simulink model "chap6_6sim"  (Simulink 7.7)
settings: Solver=ode45  StartTime=0.0  StopTime=10.0  RelTol=1e-3
settings Model: Creator=Administrator  LastModifiedBy=ljk
settings DataIOCC: SignalLoggingName=sigsOut
settings OptimizationCC: InitFltsAndDblsToZero=on
settings DebuggingCC: SaveWithParameterizedLinksMsg=none  SignalResolutionControl=TryResolveAllWithWarning  SolverPrmCheckMsg=none  MultiTaskDSMMsg=warning  MultiTaskCondExecSysMsg=none  StrictBusMsg=Warning
settings HardwareCC: TargetUnknown=on
settings RTWCC: IncludeERTFirstTime=on
settings GRTTargetCC: TargetFcnLib=ansi_tfl_tmw.mat

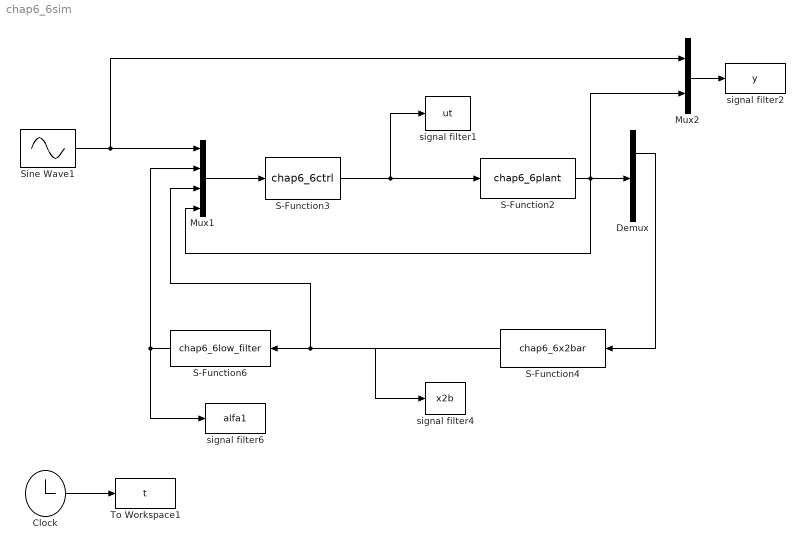
== system chap6_6sim ==
  Clock : Clock
      settings: Decimation=10
  Demux : Demux  Outputs=2
  Mux1 : Mux
  Mux2 : Mux  Inputs=2
  S-Function2 : S-Function  FunctionName=chap6_6plant  EnableBusSupport=off
  S-Function3 : S-Function  FunctionName=chap6_6ctrl  EnableBusSupport=off
  S-Function4 : S-Function  FunctionName=chap6_6x2bar  EnableBusSupport=off
  S-Function6 : S-Function  FunctionName=chap6_6low_filter  EnableBusSupport=off
  Sine Wave1 : Sin  SampleTime=0
  To Workspace1 : ToWorkspace  VariableName=t  SampleTime=-1  SaveFormat=Array
  signal filter1 : ToWorkspace  VariableName=ut  SampleTime=-1  SaveFormat=Array
  signal filter2 : ToWorkspace  VariableName=y  SampleTime=-1  SaveFormat=Array
  signal filter4 : ToWorkspace  VariableName=x2b  SampleTime=-1  SaveFormat=Array
  signal filter6 : ToWorkspace  VariableName=alfa1  SampleTime=-1  SaveFormat=Array
  wires:
  Clock/1 -> To Workspace1/1
  Mux1/1 -> S-Function3/1
  S-Function4/1 -> Mux1/3, signal filter4/1, S-Function6/1
  Sine Wave1/1 -> Mux1/1, Mux2/1
  S-Function6/1 -> Mux1/2, signal filter6/1
  S-Function2/1 -> Demux/1, Mux1/4, Mux2/2
  Demux/1 -> S-Function4/1
  Mux2/1 -> signal filter2/1
  S-Function3/1 -> S-Function2/1, signal filter1/1
